simulink model "Es1_s"  (R2014a)
settings: Solver=ode45  StartTime=0.0  StopTime=10  RelTol=1e-7
libraries: cstblocks x2, simulink x2
settings Model: Creator=Davide  LastModifiedBy=Davide

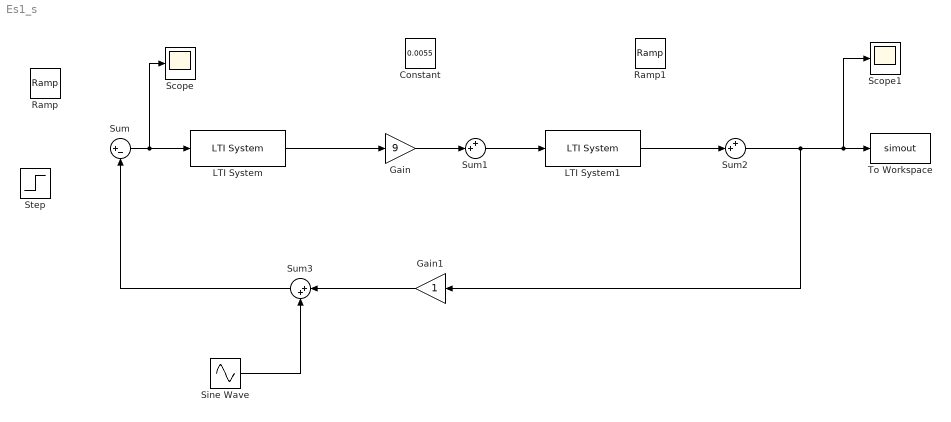
== system Es1_s ==
  Constant : Constant  Value=0.0055
  Gain : Gain  Gain=9
  Gain1 : Gain
  LTI System : cstblocks/LTI System  sys=C  IC=[]
  LTI System1 : cstblocks/LTI System  sys=Gp  IC=[]
  Ramp : simulink/Sources/Ramp  slope=1  start=0  X0=0
  Ramp1 : simulink/Sources/Ramp  slope=0.0055  start=0  X0=0
  Scope : Scope
  Scope1 : Scope
  Sine Wave : Sin  Amplitude=0.001  Frequency=30  SampleTime=0
  Step : Step  Time=0  SampleTime=0
  Sum : Sum  Inputs=|+-
  Sum1 : Sum  Inputs=++|
  Sum2 : Sum  Inputs=++|
  Sum3 : Sum  Inputs=|++
  To Workspace : ToWorkspace  VariableName=simout  SaveFormat=Timeseries  SampleTime=-1
  wires:
  Sum/1 -> Scope/1, LTI System/1
  LTI System/1 -> Gain/1
  Sum1/1 -> LTI System1/1
  Gain/1 -> Sum1/2
  LTI System1/1 -> Sum2/2
  Sum2/1 -> Gain1/1, Scope1/1, To Workspace/1
  Gain1/1 -> Sum3/1
  Sum3/1 -> Sum/2
  Sine Wave/1 -> Sum3/2
